simulink model "driver_R2023a"  (R2023a)
settings: Solver=ode5  StartTime=0.0  StopTime=inf  RelTol=1e-3
undefined symbols (not defined in the file): canChannel
libraries: canmsglib x7, canlib x5, sldrtlib x1
settings Model: Creator=nineday  LastModifiedBy=nineday
settings HardwareCC: ProdBitPerLong=64  ProdHWDeviceType=Intel->x86-64 (Linux 64)
settings ModelReferenceCC: EnableRefExpFcnMdlSchedulingChecks=on
settings RTWCC: Description=Simulink Desktop Real-Time  SystemTargetFile=sldrt.tlc  TemplateMakefile=sldrt.tmf  RTWCompilerOptimization=on
settings CodeAppCC: MaxIdLength=95
settings SimulinkDesktopRealTimeCC: TargetLibSuffix=_sldrt.a  TargetPreCompLibLocation=D:\A_Work\matlab2023\toolbox\sldrt\lib\win64

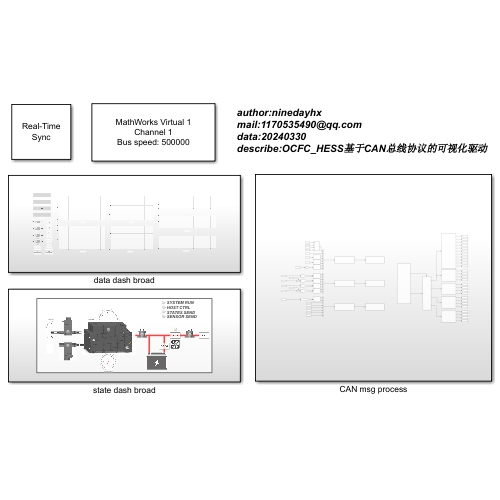
[thumbnail: Simulink's stored preview of the top-level diagram]
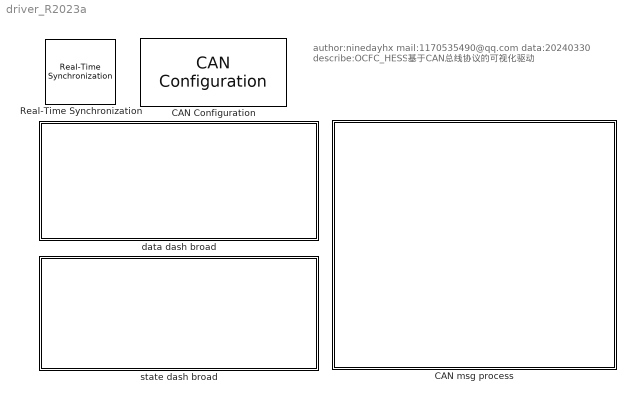
== system driver_R2023a ==
  note: author:ninedayhx
      | mail:1170535490@qq.com
      | data:20240330
      | describe:OCFC_HESS基于CAN总线协议的可视化驱动
  CAN Configuration : canlib/CAN Configuration  BlockHandle=2.0001  Device=MathWorks Virtual 1 (Channel 1)  DeviceMenu=MathWorks Virtual 1 (Channel 1)  ObjConstructor=canChannel('MathWorks', 'Virtual 1', 1)  BusSpeed=500000  EnableBitParameters=off  AckMode=Normal
  CAN msg process : Subsystem
  Real-Time Synchronization : sldrtlib/Real-Time Synchronization  SampleTime=0.01  MaxMissedTicks=100  ShowMissedTicks=off  YieldWhenWaiting=on
  data dash broad : Subsystem
  state dash broad : Subsystem

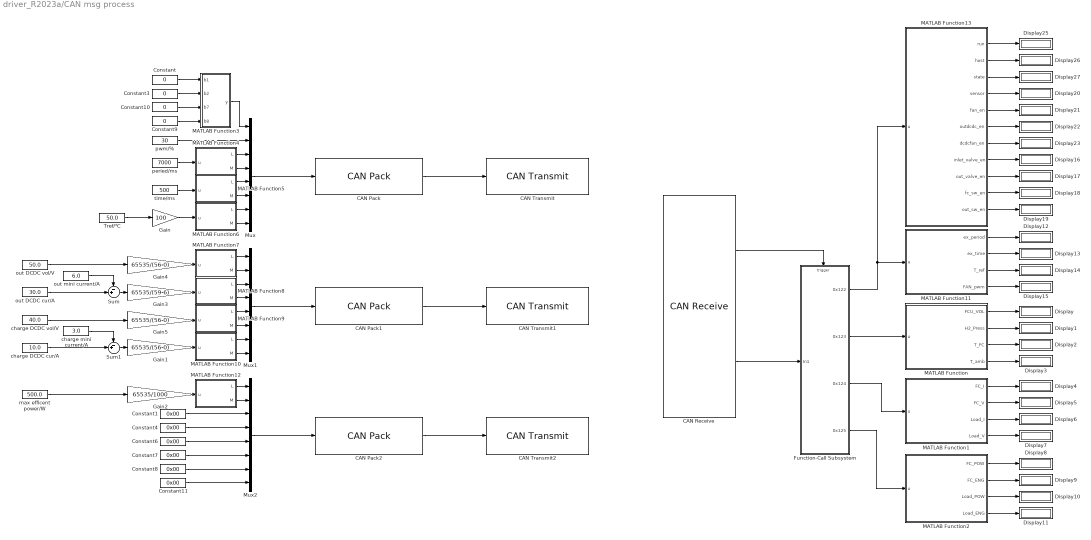
== system driver_R2023a/CAN msg process ==
  CAN Pack : canmsglib/CAN Pack  MsgList=(none)  MsgName=CAN Msg  MsgIDType=Standard (11-bit identifier)  MsgIdentifier=0x456  MsgLength=8  Remote=off  ApplyMinMax=off  BusOutput=off  SignalInfo={}
      settings: DataFormat=raw data
  CAN Pack1 : canmsglib/CAN Pack  MsgList=(none)  MsgName=CAN Msg  MsgIDType=Standard (11-bit identifier)  MsgIdentifier=0x457  MsgLength=8  Remote=off  ApplyMinMax=off  BusOutput=off  SignalInfo={}
      settings: DataFormat=raw data
  CAN Pack2 : canmsglib/CAN Pack  MsgList=(none)  MsgName=CAN Msg  MsgIDType=Standard (11-bit identifier)  MsgIdentifier=0x458  MsgLength=8  Remote=off  ApplyMinMax=off  BusOutput=off  SignalInfo={}
      settings: DataFormat=raw data
  CAN Receive : canlib/CAN Receive  BlockHandle=13.0001  Device=MathWorks Virtual 1 (Channel 1)  DeviceMenu=MathWorks Virtual 1 (Channel 1)  ObjConstructor=canChannel('MathWorks', 'Virtual 1', 1)  EnableStandardIDsFilter=off  StdIDsCombo=Allow all  StandardIDs=0  EnableExtendedIDsFilter=off  ExtIDsCombo=Allow all  ExtendedIDs=0  SampleTime=0.01  MsgsPerTimestep=all  InternalFilterUpdateStatus=on  BusOutput=off
  CAN Transmit : canlib/CAN Transmit  BlockHandle=16.0001  Device=MathWorks Virtual 1 (Channel 1)  DeviceMenu=MathWorks Virtual 1 (Channel 1)  ObjConstructor=canChannel('MathWorks', 'Virtual 1', 1)  EnableEventTransmit=on  EnablePeriodicTransmit=off  MessagePeriod=1.000
  CAN Transmit1 : canlib/CAN Transmit  BlockHandle=18.0001  Device=MathWorks Virtual 1 (Channel 1)  DeviceMenu=MathWorks Virtual 1 (Channel 1)  ObjConstructor=canChannel('MathWorks', 'Virtual 1', 1)  EnableEventTransmit=on  EnablePeriodicTransmit=off  MessagePeriod=1.000
  CAN Transmit2 : canlib/CAN Transmit  BlockHandle=20.0001  Device=MathWorks Virtual 1 (Channel 1)  DeviceMenu=MathWorks Virtual 1 (Channel 1)  ObjConstructor=canChannel('MathWorks', 'Virtual 1', 1)  EnableEventTransmit=on  EnablePeriodicTransmit=off  MessagePeriod=1.000
  Constant{,3,9..10} (4 alike) : Constant  Value=0
  Constant{1,4,6..8,11} (6 alike) : Constant  Value=0x00
  Display{,1..23,25..27} (27 alike) : Display
  Function-Call Subsystem : Subsystem  TreatAsAtomicUnit=on
  Gain : Gain  Gain=100
  Gain1 : Gain  Gain=65535/(56-0)
  Gain2 : Gain  Gain=65535/1000
  Gain3 : Gain  Gain=65535/(59-6)
  Gain4 : Gain  Gain=65535/(56-0)
  Gain5 : Gain  Gain=65535/(56-0)
  MATLAB Function : MATLAB Function  TreatAsAtomicUnit=on
  MATLAB Function1 : MATLAB Function  TreatAsAtomicUnit=on
  MATLAB Function10 : MATLAB Function  TreatAsAtomicUnit=on
  MATLAB Function11 : MATLAB Function  TreatAsAtomicUnit=on
  MATLAB Function12 : MATLAB Function  TreatAsAtomicUnit=on
  MATLAB Function13 : MATLAB Function  TreatAsAtomicUnit=on
  MATLAB Function2 : MATLAB Function  TreatAsAtomicUnit=on
  MATLAB Function3 : MATLAB Function  TreatAsAtomicUnit=on
  MATLAB Function4 : MATLAB Function  TreatAsAtomicUnit=on
  MATLAB Function5 : MATLAB Function  TreatAsAtomicUnit=on
  MATLAB Function6 : MATLAB Function  TreatAsAtomicUnit=on
  MATLAB Function7 : MATLAB Function  TreatAsAtomicUnit=on
  MATLAB Function8 : MATLAB Function  TreatAsAtomicUnit=on
  MATLAB Function9 : MATLAB Function  TreatAsAtomicUnit=on
  Mux : Mux  Inputs=8
  Mux1 : Mux  Inputs=8
  Mux2 : Mux  Inputs=8
  Sum : Sum  Inputs=-+|
  Sum1 : Sum  Inputs=-+|
  Tref/℃ : Constant  Value=50.0  OutDataTypeStr=uint8
  charge DCDC cur/A : Constant  Value=10.0  OutDataTypeStr=uint8
  charge DCDC vol/V : Constant  Value=40.0  OutDataTypeStr=uint8
  charge mini current/A : Constant  Value=3.0  OutDataTypeStr=uint8
  max efficent power/W : Constant  Value=500.0
  out DCDC cur/A : Constant  Value=30.0  OutDataTypeStr=uint8
  out DCDC vol/V : Constant  Value=50.0  OutDataTypeStr=uint8
  out mini current/A : Constant  Value=6.0  OutDataTypeStr=uint8
  peried/ms : Constant  Value=7000  OutDataTypeStr=uint8
  pwm/% : Constant  Value=30  OutDataTypeStr=uint8
  time/ms : Constant  Value=500  OutDataTypeStr=uint8
  wires:
  MATLAB Function5/2(M) -> Mux/6
  MATLAB Function4/2(M) -> Mux/4
  MATLAB Function1/2(FC_V) -> Display5/1
  CAN Pack/1 -> CAN Transmit/1
  MATLAB Function5/1(L) -> Mux/5
  MATLAB Function1/1(FC_I) -> Display4/1
  CAN Receive/1 -> Function-Call Subsystem/Trigger
  MATLAB Function1/4(Load_V) -> Display7/1
  MATLAB Function/3(T_FC) -> Display2/1
  MATLAB Function/4(T_amb) -> Display3/1
  MATLAB Function3/1(y) -> Mux/1
  CAN Receive/2 -> Function-Call Subsystem/1(In1)
  MATLAB Function/2(H2_Press) -> Display1/1
  Function-Call Subsystem/4(0x125) -> MATLAB Function2/1(u)
  Function-Call Subsystem/2(0x123) -> MATLAB Function/1(u)
  MATLAB Function2/1(FC_POW) -> Display8/1
  Function-Call Subsystem/3(0x124) -> MATLAB Function1/1(u)
  MATLAB Function6/1(L) -> Mux/7
  MATLAB Function4/1(L) -> Mux/3
  MATLAB Function/1(FCU_VOL) -> Display/1
  MATLAB Function2/2(FC_ENG) -> Display9/1
  pwm/%/1 -> Mux/2
  MATLAB Function6/2(M) -> Mux/8
  MATLAB Function2/3(Load_POW) -> Display10/1
  MATLAB Function2/4(Load_ENG) -> Display11/1
  MATLAB Function1/3(Load_I) -> Display6/1
  Mux/1 -> CAN Pack/1
  Constant/1 -> MATLAB Function3/1(b1)
  Constant9/1 -> MATLAB Function3/4(b8)
  Constant3/1 -> MATLAB Function3/2(b2)
  Constant10/1 -> MATLAB Function3/3(b7)
  peried/ms/1 -> MATLAB Function4/1(u)
  time/ms/1 -> MATLAB Function5/1(u)
  Tref/℃/1 -> Gain/1
  Gain/1 -> MATLAB Function6/1(u)
  Gain5/1 -> MATLAB Function9/1(u)
  MATLAB Function9/1(L) -> Mux1/5
  MATLAB Function8/2(M) -> Mux1/4
  MATLAB Function9/2(M) -> Mux1/6
  MATLAB Function10/2(M) -> Mux1/8
  Gain3/1 -> MATLAB Function8/1(u)
  MATLAB Function8/1(L) -> Mux1/3
  Mux1/1 -> CAN Pack1/1
  MATLAB Function10/1(L) -> Mux1/7
  CAN Pack1/1 -> CAN Transmit1/1
  Gain1/1 -> MATLAB Function10/1(u)
  CAN Pack2/1 -> CAN Transmit2/1
  Constant6/1 -> Mux2/5
  Mux2/1 -> CAN Pack2/1
  Constant11/1 -> Mux2/8
  Constant7/1 -> Mux2/6
  Constant4/1 -> Mux2/4
  Constant8/1 -> Mux2/7
  Constant1/1 -> Mux2/3
  MATLAB Function7/1(L) -> Mux1/1
  MATLAB Function7/2(M) -> Mux1/2
  Gain4/1 -> MATLAB Function7/1(u)
  out DCDC vol/V/1 -> Gain4/1
  out DCDC cur/A/1 -> Sum/2
  Sum/1 -> Gain3/1
  out mini current/A/1 -> Sum/1
  charge DCDC vol/V/1 -> Gain5/1
  charge DCDC cur/A/1 -> Sum1/2
  charge mini current/A/1 -> Sum1/1
  Sum1/1 -> Gain1/1
  MATLAB Function12/1(L) -> Mux2/1
  MATLAB Function12/2(M) -> Mux2/2
  Gain2/1 -> MATLAB Function12/1(u)
  max efficent power/W/1 -> Gain2/1
  Function-Call Subsystem/1(0x122) -> MATLAB Function13/1(u), MATLAB Function11/1(u)
  MATLAB Function11/1(ex_period) -> Display12/1
  MATLAB Function11/2(ex_time) -> Display13/1
  MATLAB Function11/3(T_ref) -> Display14/1
  MATLAB Function11/4(FAN_pwm) -> Display15/1
  MATLAB Function13/1(run) -> Display25/1
  MATLAB Function13/2(host) -> Display26/1
  MATLAB Function13/3(state) -> Display27/1
  MATLAB Function13/4(sensor) -> Display20/1
  MATLAB Function13/5(fan_en) -> Display21/1
  MATLAB Function13/6(outdcdc_en) -> Display22/1
  MATLAB Function13/7(dcdcfan_en) -> Display23/1
  MATLAB Function13/8(inlet_valve_en) -> Display16/1
  MATLAB Function13/9(out_valve_en) -> Display17/1
  MATLAB Function13/10(fc_sw_en) -> Display18/1
  MATLAB Function13/11(out_sw_en) -> Display19/1

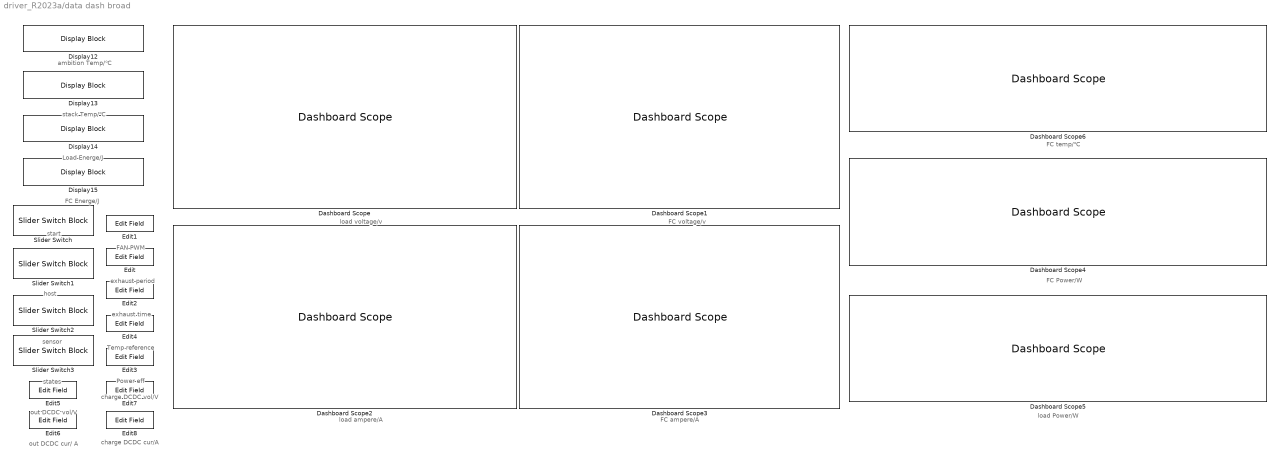
== system driver_R2023a/data dash broad ==
  note: load voltage/v
  note: load ampere/A
  note: FC voltage/v
  note: FC ampere/A
  note: FC Power/W
  note: load Power/W
  note: ambition Temp/℃
  note: stack Temp/℃
  note: Load Energe/J
  note: FC Energe/J
  note: FC temp/℃
  note: start
  note: host
  note: sensor
  note: exhaust period
  note: FAN PWM
  note: exhaust time
  note: states
  note: Temp reference
  note: Power eff
  note: out DCDC vol/V
  note: out DCDC cur/ A
  note: charge DCDC vol/V
  note: charge DCDC cur/A
  Dashboard Scope : DashboardScope  ShowInitialText=off  Ymin=48  Ymax=52  ScaleAtStop=off  UpdateMode=Scroll
      settings: TickLabels=Y-Axis
  Dashboard Scope1 : DashboardScope  ShowInitialText=off  Ymin=0  Ymax=50  ScaleAtStop=off  UpdateMode=Scroll  Markers=on
      settings: TickLabels=Y-Axis
  Dashboard Scope2 : DashboardScope  ShowInitialText=off  Ymin=0  Ymax=25  ScaleAtStop=off  UpdateMode=Scroll
      settings: TickLabels=Y-Axis
  Dashboard Scope3 : DashboardScope  ShowInitialText=off  Ymin=0  Ymax=30  ScaleAtStop=off  UpdateMode=Scroll  Markers=on
      settings: TickLabels=Y-Axis
  Dashboard Scope4 : DashboardScope  ShowInitialText=off  Ymin=0  Ymax=1000  ScaleAtStop=off  UpdateMode=Scroll
      settings: TickLabels=Y-Axis
  Dashboard Scope5 : DashboardScope  ShowInitialText=off  Ymin=0  Ymax=1500  ScaleAtStop=off
      settings: TickLabels=Y-Axis
  Dashboard Scope6 : DashboardScope  ShowInitialText=off  Ymin=0  Ymax=60  ScaleAtStop=off  UpdateMode=Scroll
      settings: TickLabels=Y-Axis
  Display{12..15} (4 alike) : DisplayBlock  LabelPosition=Hide  Transparency=1
  Edit{,1..8} (9 alike) : EditField  LabelPosition=Hide  ShowInitialText=on  Alignment=Center
  Slider Switch{,1..3} (4 alike) : SliderSwitchBlock  LabelPosition=Hide
      settings: Values={{'Off', 'On'}, [0 1]}

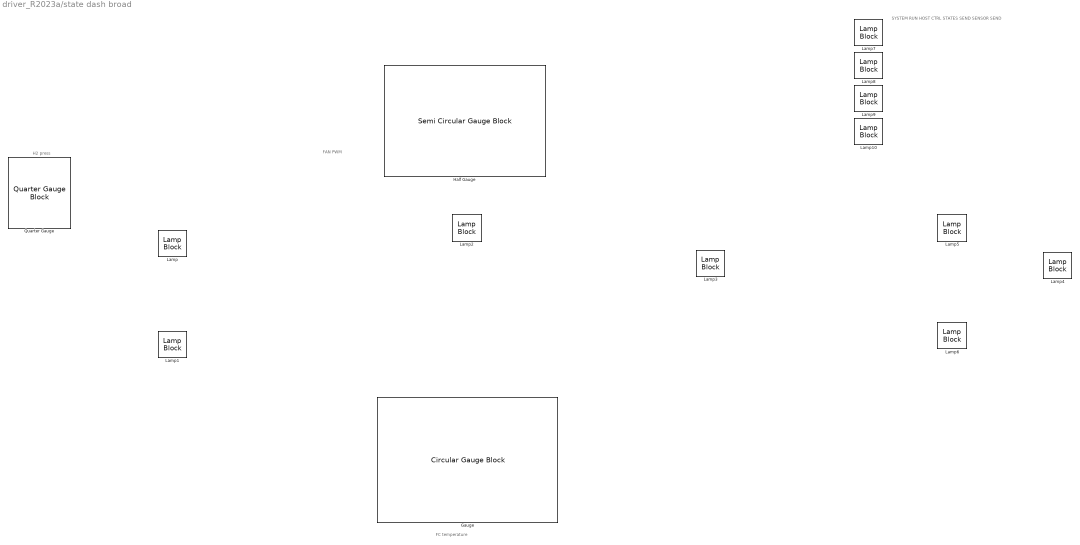
== system driver_R2023a/state dash broad ==
  note: H2 press
  note: SYSTEM RUN
      | HOST CTRL
      | STATES SEND
      | SENSOR SEND
  note: FAN PWM
  note: FC temperature
  Gauge : CircularGaugeBlock  LabelPosition=Hide
  Half Gauge : SemiCircularGaugeBlock  LabelPosition=Hide
  Lamp{,1..10} (11 alike) : LampBlock  LabelPosition=Hide
  Quarter Gauge : QuarterGaugeBlock  LabelPosition=Hide  ScaleMax=20

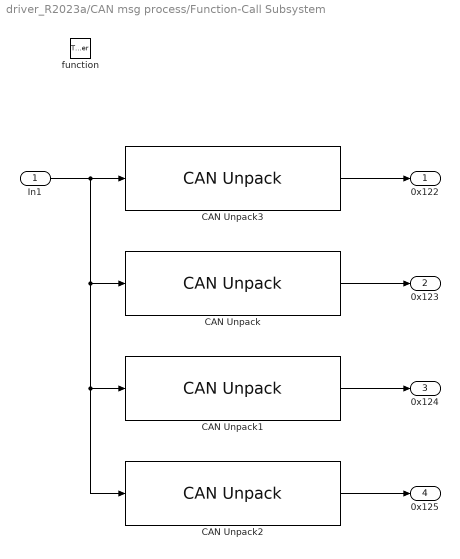
== system driver_R2023a/CAN msg process/Function-Call Subsystem ==
  In1 : Inport
  function : TriggerPort  TriggerType=function-call  VariantControl=(inherit)
  CAN Unpack : canmsglib/CAN Unpack  MsgList=(none)  MsgName=CAN Msg  MsgIDType=Standard (11-bit identifier)  MsgIdentifier=0x123  MsgLength=8  SignalInfo={}  IDPort=off  TimestampPort=off  ErrorPort=off  RemotePort=off  LengthPort=off  StatusPort=off  ApplyMinMax=off
      settings: DataFormat=raw data
  CAN Unpack1 : canmsglib/CAN Unpack  MsgList=(none)  MsgName=CAN Msg  MsgIDType=Standard (11-bit identifier)  MsgIdentifier=0x124  MsgLength=8  SignalInfo={}  IDPort=off  TimestampPort=off  ErrorPort=off  RemotePort=off  LengthPort=off  StatusPort=off  ApplyMinMax=off
      settings: DataFormat=raw data
  CAN Unpack2 : canmsglib/CAN Unpack  MsgList=(none)  MsgName=CAN Msg  MsgIDType=Standard (11-bit identifier)  MsgIdentifier=0x125  MsgLength=8  SignalInfo={}  IDPort=off  TimestampPort=off  ErrorPort=off  RemotePort=off  LengthPort=off  StatusPort=off  ApplyMinMax=off
      settings: DataFormat=raw data
  CAN Unpack3 : canmsglib/CAN Unpack  MsgList=(none)  MsgName=CAN Msg  MsgIDType=Standard (11-bit identifier)  MsgIdentifier=0x122  MsgLength=8  SignalInfo={}  IDPort=off  TimestampPort=off  ErrorPort=off  RemotePort=off  LengthPort=off  StatusPort=off  ApplyMinMax=off
      settings: DataFormat=raw data
  0x122 : Outport
  0x123 : Outport  Port=2
  0x124 : Outport  Port=3
  0x125 : Outport  Port=4
  wires:
  In1/1 -> CAN Unpack2/1, CAN Unpack1/1, CAN Unpack/1, CAN Unpack3/1
  CAN Unpack/1 -> 0x123/1
  CAN Unpack1/1 -> 0x124/1
  CAN Unpack2/1 -> 0x125/1
  CAN Unpack3/1 -> 0x122/1

== matlab function driver_R2023a/CAN msg process/MATLAB Function9 ==
  data: L output; u input; M output
function [L, M]= fcn(u)
u1 = uint16(u);
M = uint8(u1);
L = bitshift(u1,-8);

== matlab function driver_R2023a/CAN msg process/MATLAB Function11 ==
  data: u input; ex_period output; ex_time output; T_ref output; FAN_pwm output
function [ex_period, ex_time, T_ref, FAN_pwm] = fcn(u)
ex_period = bitshift(uint16(u(3)),8) + uint16(u(4));
ex_time =  bitshift(uint16(u(5)),8) + uint16(u(6));
T_ref =  bitshift(uint16(u(7)),2) + uint16(bitand(u(8),0x03));
FAN_pwm = bitshift(u(8),-2);

== matlab function driver_R2023a/CAN msg process/MATLAB Function12 ==
  data: L output; u input; M output
function [L, M]= fcn(u)
u1 = uint16(u);
M = uint8(u1);
L = bitshift(u1,-8);

== matlab function driver_R2023a/CAN msg process/MATLAB Function13 ==
  data: u input; run output; host output; state output; sensor output; fan_en output; outdcdc_en output; dcdcfan_en output; inlet_valve_en output; out_valve_en output; fc_sw_en output; out_sw_en output
function [run, host, state, sensor, fan_en, outdcdc_en, dcdcfan_en, inlet_valve_en, out_valve_en, fc_sw_en, out_sw_en] = fcn(u)
run = bitget(u(1),2);
host = bitget(u(1),6);
state = bitget(u(1),7);
sensor = bitget(u(1),8);
fan_en = bitget(u(2),1);
outdcdc_en = bitget(u(2),2);
dcdcfan_en = bitget(u(2),3);
inlet_valve_en = bitget(u(2),4);
out_valve_en = bitget(u(2),5);
fc_sw_en = bitget(u(2),6);
out_sw_en = bitget(u(2),7);

== matlab function driver_R2023a/CAN msg process/MATLAB Function1 ==
  data: u input; FC_I output; FC_V output; Load_I output; Load_V output
function [FC_I, FC_V, Load_I, Load_V] = fcn(u)
FC_I = hex2dec([dec2hex(u(1)), dec2hex(u(2))])/100;
FC_V = hex2dec([dec2hex(u(3)), dec2hex(u(4))])/100;
Load_I = hex2dec([dec2hex(u(5)), dec2hex(u(6))])/100;
Load_V = hex2dec([dec2hex(u(7)), dec2hex(u(8))])/100;

== matlab function driver_R2023a/CAN msg process/MATLAB Function ==
  data: u input; FCU_VOL output; H2_Press output; T_FC output; T_amb output
function [FCU_VOL, H2_Press, T_FC, T_amb] = fcn(u)
FCU_VOL = hex2dec([dec2hex(u(1)), dec2hex(u(2))])/100;
H2_Press = hex2dec([dec2hex(u(3)), dec2hex(u(4))])/100;
T_FC = hex2dec([dec2hex(u(5)), dec2hex(u(6))])/100;
T_amb = hex2dec([dec2hex(u(7)), dec2hex(u(8))])/100;

== matlab function driver_R2023a/CAN msg process/MATLAB Function2 ==
  data: u input; FC_POW output; FC_ENG output; Load_POW output; Load_ENG output
function [FC_POW, FC_ENG, Load_POW, Load_ENG] = fcn(u)
FC_POW = hex2dec([dec2hex(u(1)), dec2hex(u(2))])/100;
FC_ENG = hex2dec([dec2hex(u(3)), dec2hex(u(4))])/100;
Load_POW = hex2dec([dec2hex(u(5)), dec2hex(u(6))])/100;
Load_ENG = hex2dec([dec2hex(u(7)), dec2hex(u(8))])/100;

== matlab function driver_R2023a/CAN msg process/MATLAB Function3 ==
  data: b1 input; y output; b2 input; b7 input; b8 input
function y = fcn(b1,b2,b7,b8)
z=b1+2*b2+2^6*b7+2^7*b8;
y = uint8(z);

== matlab function driver_R2023a/CAN msg process/MATLAB Function4 ==
  data: L output; u input; M output
function [L, M]= fcn(u)
u1 = uint16(u);
M = uint8(u1);
L = bitshift(u1,-8);

== matlab function driver_R2023a/CAN msg process/MATLAB Function5 ==
  data: L output; u input; M output
function [L, M]= fcn(u)
u1 = uint16(u);
M = uint8(u1);
L = bitshift(u1,-8);

== matlab function driver_R2023a/CAN msg process/MATLAB Function6 ==
  data: L output; u input; M output
function [L, M]= fcn(u)
u1 = uint16(u);
M = uint8(u1);
L = bitshift(u1,-8);

== matlab function driver_R2023a/CAN msg process/MATLAB Function10 ==
  data: L output; u input; M output
function [L, M]= fcn(u)
u1 = uint16(u);
M = uint8(u1);
L = bitshift(u1,-8);

== matlab function driver_R2023a/CAN msg process/MATLAB Function7 ==
  data: L output; u input; M output
function [L, M]= fcn(u)
u1 = uint16(u);
M = uint8(u1);
L = bitshift(u1,-8);

== matlab function driver_R2023a/CAN msg process/MATLAB Function8 ==
  data: L output; u input; M output
function [L, M]= fcn(u)
u1 = uint16(u);
M = uint8(u1);
L = bitshift(u1,-8);
